simulink model "RM3_cHydraulic_PTO_WithSimscapeJustPiston"  (R2020b)
settings: Solver=ode4  StartTime=0  StopTime=400  FixedStep=0.001  MaxStep=0.001  RelTol=1e-3
values from neighbouring files (symbols this model uses):
  Apiston = 0.0378    [ptoSimInputFile.m]
  Vo_cylinder = 15*Apiston    (= 0.567)    [ptoSimInputFile.m]
undefined symbols (not defined in the file or in its folder): RM3_CHydraulic_resultsOriginal
libraries: fl_lib x13, nesl_utility x8, PTOSim_Lib x2, sh_lib x1
settings Model: Creator=jleonqu  LastModifiedBy=jleonqu
settings SolverCC: ZeroCrossControl=DisableAll  AutoInsertRateTranBlk=on
settings DataIOCC: ReturnWorkspaceOutputs=off
settings OptimizationCC: SimCompilerOptimization=on

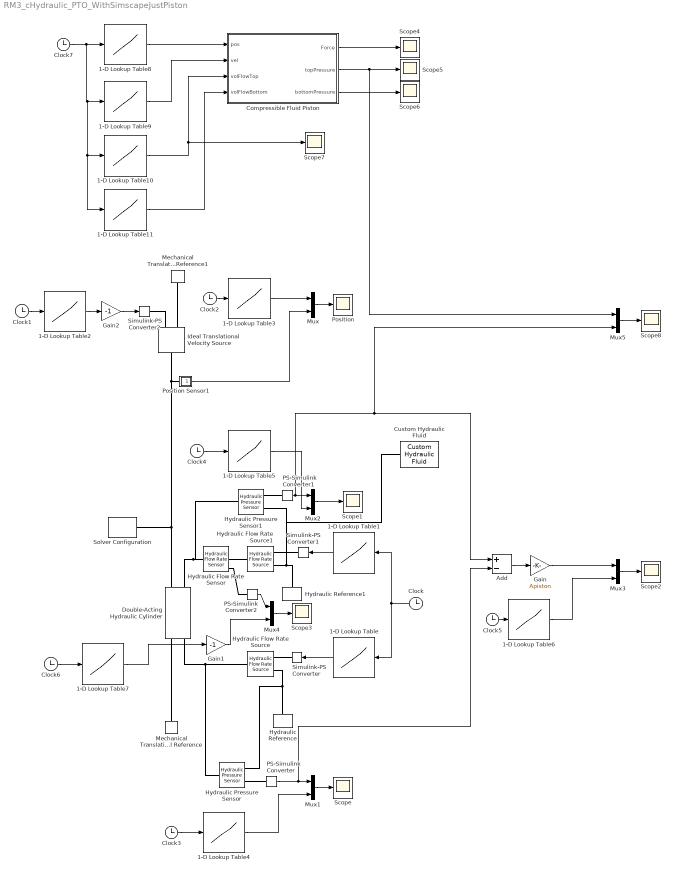
== system RM3_cHydraulic_PTO_WithSimscapeJustPiston ==
  1-D Lookup Table : Lookup_n-D  NumberOfTableDimensions=1  BreakpointsForDimension1=RM3_CHydraulic_resultsOriginal(:,1)  Table=RM3_CHydraulic_resultsOriginal(:,5)  InternalRulePriority=Speed  RndMeth=Simplest  InputSameDT=on
  1-D Lookup Table1 : Lookup_n-D  NumberOfTableDimensions=1  BreakpointsForDimension1=RM3_CHydraulic_resultsOriginal(:,1)  Table=RM3_CHydraulic_resultsOriginal(:,4)  InternalRulePriority=Speed  RndMeth=Simplest  InputSameDT=on
  1-D Lookup Table10 : Lookup_n-D  NumberOfTableDimensions=1  BreakpointsForDimension1=RM3_CHydraulic_resultsOriginal(:,1)  Table=RM3_CHydraulic_resultsOriginal(:,4)  InternalRulePriority=Speed  RndMeth=Simplest  InputSameDT=on
  1-D Lookup Table11 : Lookup_n-D  NumberOfTableDimensions=1  BreakpointsForDimension1=RM3_CHydraulic_resultsOriginal(:,1)  Table=RM3_CHydraulic_resultsOriginal(:,5)  InternalRulePriority=Speed  RndMeth=Simplest  InputSameDT=on
  1-D Lookup Table2 : Lookup_n-D  NumberOfTableDimensions=1  BreakpointsForDimension1=RM3_CHydraulic_resultsOriginal(:,1)  Table=RM3_CHydraulic_resultsOriginal(:,3)  InternalRulePriority=Speed  RndMeth=Simplest  InputSameDT=on
  1-D Lookup Table3 : Lookup_n-D  NumberOfTableDimensions=1  BreakpointsForDimension1=RM3_CHydraulic_resultsOriginal(:,1)  Table=RM3_CHydraulic_resultsOriginal(:,2)  InternalRulePriority=Speed  RndMeth=Simplest  InputSameDT=on
  1-D Lookup Table4 : Lookup_n-D  NumberOfTableDimensions=1  BreakpointsForDimension1=RM3_CHydraulic_resultsOriginal(:,1)  Table=RM3_CHydraulic_resultsOriginal(:,8)  InternalRulePriority=Speed  RndMeth=Simplest  InputSameDT=on
  1-D Lookup Table5 : Lookup_n-D  NumberOfTableDimensions=1  BreakpointsForDimension1=RM3_CHydraulic_resultsOriginal(:,1)  Table=RM3_CHydraulic_resultsOriginal(:,7)  InternalRulePriority=Speed  RndMeth=Simplest  InputSameDT=on
  1-D Lookup Table6 : Lookup_n-D  NumberOfTableDimensions=1  BreakpointsForDimension1=RM3_CHydraulic_resultsOriginal(:,1)  Table=RM3_CHydraulic_resultsOriginal(:,6)  InternalRulePriority=Speed  RndMeth=Simplest  InputSameDT=on
  1-D Lookup Table7 : Lookup_n-D  NumberOfTableDimensions=1  BreakpointsForDimension1=RM3_CHydraulic_resultsOriginal(:,1)  Table=RM3_CHydraulic_resultsOriginal(:,4)  InternalRulePriority=Speed  RndMeth=Simplest  InputSameDT=on
  1-D Lookup Table8 : Lookup_n-D  NumberOfTableDimensions=1  BreakpointsForDimension1=RM3_CHydraulic_resultsOriginal(:,1)  Table=RM3_CHydraulic_resultsOriginal(:,2)  InternalRulePriority=Speed  RndMeth=Simplest  InputSameDT=on
  1-D Lookup Table9 : Lookup_n-D  NumberOfTableDimensions=1  BreakpointsForDimension1=RM3_CHydraulic_resultsOriginal(:,1)  Table=RM3_CHydraulic_resultsOriginal(:,3)  InternalRulePriority=Speed  RndMeth=Simplest  InputSameDT=on
  Add : Sum  Inputs=+-
  Clock{,1..7} (8 alike) : Clock
  Compressible Fluid Piston : Subsystem
  Custom Hydraulic Fluid : fl_lib/Hydraulic/Hydraulic Utilities/Custom Hydraulic Fluid  density=850 kg/m^3  viscosity_kin=18e-6 m^2/s  bulk=1.86e9 Pa  alpha=0.005  range_error=2
      settings: SourceProductBaseCode=SS  InternalSimscapePortConfiguration="{\"Bottom\":[],\"Left\":[],\"Right\":[{\"id\":\"G\",\"label\":\"\",\"type\":\"foundation.hydraulic.hydraulic\"}],\"Top\":[]}"
  Double-Acting Hydraulic Cylinder : sh_lib/Hydraulic Cylinders/Double-Acting Hydraulic Cylinder  area_A=Apiston m^2  area_B=Apiston m^2  stroke=2*Vo_cylinder/Apiston m  init_pos=0.3*2*Vo_cylinder/Apiston m  dead_vol_A=1e-4 m^3  dead_vol_B=1e-4 m^3  init_pressure_A=2.1333e7 Pa  init_pressure_B=2.1333e7 Pa  k_sh=1.4  stiff=1e6 N/m  D=150 N/(m/s)  hardstop_model=1  transition=0.1 mm  or=1
      settings: SourceProductBaseCode=SH  InternalSimscapePortConfiguration="{\"Bottom\":[],\"Left\":[{\"id\":\"C\",\"label\":\"C\",\"type\":\"foundation.mechanical.translational.translational\"},{\"id\":\"A\",\"label\":\"A\",\"type\":\"foundation.hydraulic.hydraulic\"}],\"Right\":[{\"id\":\"R\",\"label\":\"R\",\"type\":\"foundation.mechanical.translational.translational\"},{\"id\":\"B\",\"label\":\"B\",\"type\":\"foundation.hydraulic.hydraulic\"}],\"Top\":[]}"
  Gain : Gain  Gain=Apiston
  Gain1 : Gain  Gain=-1
  Gain2 : Gain  Gain=-1
  Hydraulic Flow Rate Sensor : fl_lib/Hydraulic/Hydraulic Sensors/Hydraulic Flow Rate Sensor
  Hydraulic Flow Rate Source : fl_lib/Hydraulic/Hydraulic Sources/Hydraulic Flow Rate Source
      settings: SourceProductBaseCode=SS  InternalSimscapePortConfiguration="{\"Bottom\":[],\"Left\":[{\"id\":\"P\",\"label\":\"P\",\"type\":\"foundation.hydraulic.hydraulic\"}],\"Right\":[{\"id\":\"S\",\"label\":\"S\",\"type\":\"input\"},{\"id\":\"T\",\"label\":\"T\",\"type\":\"foundation.hydraulic.hydraulic\"}],\"Top\":[]}"
  Hydraulic Flow Rate Source1 : fl_lib/Hydraulic/Hydraulic Sources/Hydraulic Flow Rate Source
      settings: SourceProductBaseCode=SS  InternalSimscapePortConfiguration="{\"Bottom\":[],\"Left\":[{\"id\":\"P\",\"label\":\"P\",\"type\":\"foundation.hydraulic.hydraulic\"}],\"Right\":[{\"id\":\"S\",\"label\":\"S\",\"type\":\"input\"},{\"id\":\"T\",\"label\":\"T\",\"type\":\"foundation.hydraulic.hydraulic\"}],\"Top\":[]}"
  Hydraulic Pressure Sensor : fl_lib/Hydraulic/Hydraulic Sensors/Hydraulic Pressure Sensor
  Hydraulic Pressure Sensor1 : fl_lib/Hydraulic/Hydraulic Sensors/Hydraulic Pressure Sensor
  Hydraulic Reference : fl_lib/Hydraulic/Hydraulic Elements/Hydraulic Reference
  Hydraulic Reference1 : fl_lib/Hydraulic/Hydraulic Elements/Hydraulic Reference
  Ideal Translational Velocity Source : fl_lib/Mechanical/Mechanical Sources/Ideal Translational Velocity Source
  Mechanical Translational Reference : fl_lib/Mechanical/Translational Elements/Mechanical Translational Reference
  Mechanical Translational Reference1 : fl_lib/Mechanical/Translational Elements/Mechanical Translational Reference
  Mux{,1..5} (6 alike) : Mux  Inputs=2
  PS-Simulink Converter : nesl_utility/PS-Simulink Converter  PhysicalDomain=network_engine_domain  SubClassName=ps_output  LeftPortType=input  RightPortType=output  PseudoPeriodic=off  Frequencies=[]  Unit=inherit  AffineConversion=off
  PS-Simulink Converter1 : nesl_utility/PS-Simulink Converter  PhysicalDomain=network_engine_domain  SubClassName=ps_output  LeftPortType=input  RightPortType=output  PseudoPeriodic=off  Frequencies=[]  Unit=inherit  AffineConversion=off
  PS-Simulink Converter2 : nesl_utility/PS-Simulink Converter  PhysicalDomain=network_engine_domain  SubClassName=ps_output  LeftPortType=input  RightPortType=output  PseudoPeriodic=off  Frequencies=[]  Unit=inherit  AffineConversion=off
  Position : Scope
  Position Sensor1 : Subsystem
      mask Display: disp('P');
  Scope{,1..8} (9 alike) : Scope
  Simulink-PS Converter : nesl_utility/Simulink-PS Converter  PhysicalDomain=network_engine_domain  SubClassName=ps_input  LeftPortType=input  RightPortType=output  PseudoPeriodic=off  Frequencies=[]  NoiseDistribution=none  NoiseParameters=[]  Unit=1  AffineConversion=off  FilteringAndDerivatives=provide  SimscapeFilterOrder=1  InputFilterTimeConstant=0.001  UdotUserProvided=0
  Simulink-PS Converter1 : nesl_utility/Simulink-PS Converter  PhysicalDomain=network_engine_domain  SubClassName=ps_input  LeftPortType=input  RightPortType=output  PseudoPeriodic=off  Frequencies=[]  NoiseDistribution=none  NoiseParameters=[]  Unit=1  AffineConversion=off  FilteringAndDerivatives=provide  SimscapeFilterOrder=1  InputFilterTimeConstant=0.001  UdotUserProvided=0
  Simulink-PS Converter2 : nesl_utility/Simulink-PS Converter  PhysicalDomain=network_engine_domain  SubClassName=ps_input  LeftPortType=input  RightPortType=output  PseudoPeriodic=off  Frequencies=[]  NoiseDistribution=none  NoiseParameters=[]  Unit=1  AffineConversion=off  FilteringAndDerivatives=provide  SimscapeFilterOrder=1  InputFilterTimeConstant=0.001  UdotUserProvided=0
  Solver Configuration : nesl_utility/Solver Configuration  PhysicalDomain=network_engine_domain  SubClassName=solver  LeftPortType=input  RightPortType=generic  Tones=[]  Harmonics=[]  SimulateNoise=off  Profile=off  UseLocalSampling=off  EnableSwitchedLinearOptims=on  FrequencyDomain=off  UseCCode=off  RelTol=0.001  AbsTol=1e-06  MinStep=1e-09  ToWorkspace=off  RevertToSquareIcSolve=off  NumHomotopyIterations=100  PhasorMode=off  PhasorModeNumHarmonics=1  DoDC=off  ResidualTolerance=1e-09  UseLocalSolver=on  LocalSolverChoice=NE_BACKWARD_EULER_ADVANCER  LocalSolverSampleTime=0.001  DoFixedCost=on  MaxNonlinIter=3  MaxModeIter=2  ComputeImpulses=off  ImpulseIterations=2  LinearAlgebra=auto  EquationFormulation=NE_TIME_EF  DelaysMemoryBudget=1024  AutomaticFiltering=on  FilteringTimeConstant=0.001  PartitionStorageMethod=AS_NEEDED  PartitionMemoryBudget=1024  PartitionMethod=ROBUST
  wires:
  1-D Lookup Table/1 -> Simulink-PS Converter/1
  1-D Lookup Table1/1 -> Simulink-PS Converter1/1
  Clock/1 -> 1-D Lookup Table1/1, 1-D Lookup Table/1
  Clock1/1 -> 1-D Lookup Table2/1
  Clock2/1 -> 1-D Lookup Table3/1
  Mux/1 -> Position/1
  Position Sensor1/1(P) -> Mux/2
  1-D Lookup Table3/1 -> Mux/1
  PS-Simulink Converter/1 -> Add/2, Mux1/1
  1-D Lookup Table4/1 -> Mux1/2
  Mux1/1 -> Scope/1
  Clock3/1 -> 1-D Lookup Table4/1
  PS-Simulink Converter1/1 -> Mux5/2, Add/1, Mux2/1
  Clock4/1 -> 1-D Lookup Table5/1
  1-D Lookup Table5/1 -> Mux2/2
  Mux2/1 -> Scope1/1
  Add/1 -> Gain/1
  Clock5/1 -> 1-D Lookup Table6/1
  1-D Lookup Table6/1 -> Mux3/2
  Gain/1 -> Mux3/1
  Mux3/1 -> Scope2/1
  PS-Simulink Converter2/1 -> Mux4/1
  Mux4/1 -> Scope3/1
  Clock6/1 -> 1-D Lookup Table7/1
  1-D Lookup Table7/1 -> Gain1/1
  Gain1/1 -> Mux4/2
  1-D Lookup Table8/1 -> Compressible Fluid Piston/1(pos)
  1-D Lookup Table9/1 -> Compressible Fluid Piston/2(vel)
  Clock7/1 -> 1-D Lookup Table11/1, 1-D Lookup Table10/1, 1-D Lookup Table9/1, 1-D Lookup Table8/1
  1-D Lookup Table10/1 -> Scope7/1, Compressible Fluid Piston/3(volFlowTop)
  1-D Lookup Table11/1 -> Compressible Fluid Piston/4(volFlowBottom)
  Compressible Fluid Piston/1(Force) -> Scope4/1
  Compressible Fluid Piston/2(topPressure) -> Mux5/1, Scope5/1
  Compressible Fluid Piston/3(bottomPressure) -> Scope6/1
  Mux5/1 -> Scope8/1
  1-D Lookup Table2/1 -> Gain2/1
  Gain2/1 -> Simulink-PS Converter2/1
  connections:
  Hydraulic Flow Rate Source/LConn1 -- Hydraulic Pressure Sensor/LConn1 -- Double-Acting Hydraulic Cylinder/LConn2
  Hydraulic Pressure Sensor1/LConn1 -- Hydraulic Flow Rate Sensor/LConn1 -- Double-Acting Hydraulic Cylinder/RConn2
  Hydraulic Reference/LConn1 -- Hydraulic Flow Rate Source/RConn2 -- Hydraulic Pressure Sensor/RConn1
  Hydraulic Reference1/LConn1 -- Custom Hydraulic Fluid/RConn1 -- Hydraulic Pressure Sensor1/RConn1 -- Hydraulic Flow Rate Source1/RConn2
  Simulink-PS Converter/RConn1 -- Hydraulic Flow Rate Source/RConn1
  Simulink-PS Converter1/RConn1 -- Hydraulic Flow Rate Source1/RConn1
  Mechanical Translational Reference/LConn1 -- Double-Acting Hydraulic Cylinder/LConn1
  Ideal Translational Velocity Source/LConn1 -- Solver Configuration/RConn1 -- Double-Acting Hydraulic Cylinder/RConn1 -- Position Sensor1/LConn1
  Mechanical Translational Reference1/LConn1 -- Ideal Translational Velocity Source/RConn2
  Simulink-PS Converter2/RConn1 -- Ideal Translational Velocity Source/RConn1
  PS-Simulink Converter/LConn1 -- Hydraulic Pressure Sensor/RConn2
  PS-Simulink Converter1/LConn1 -- Hydraulic Pressure Sensor1/RConn2
  Hydraulic Flow Rate Sensor/RConn2 -- Hydraulic Flow Rate Source1/LConn1
  PS-Simulink Converter2/LConn1 -- Hydraulic Flow Rate Sensor/RConn1

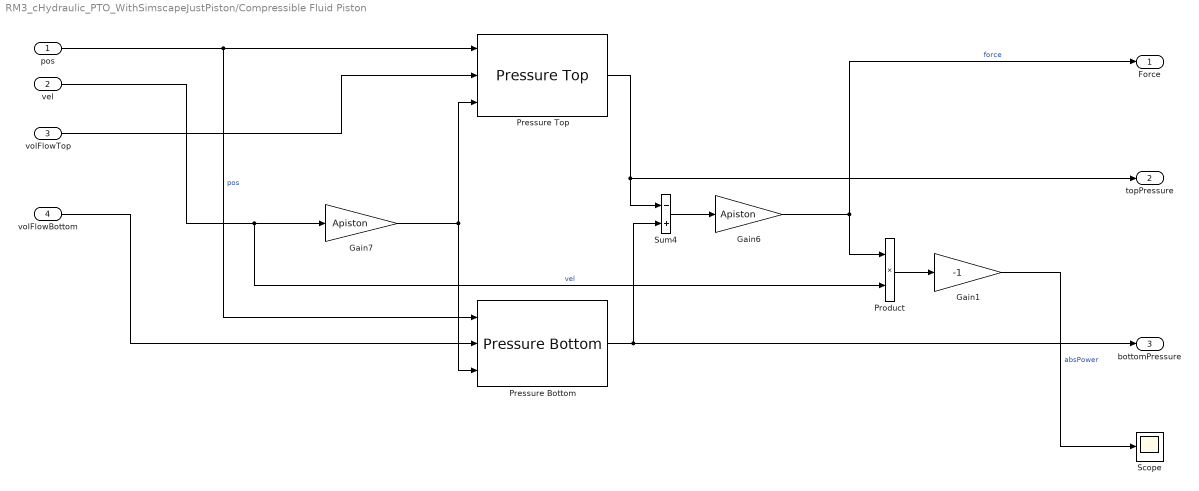
== system RM3_cHydraulic_PTO_WithSimscapeJustPiston/Compressible Fluid Piston ==
  pos : Inport
  vel : Inport  Port=2
  volFlowTop : Inport  Port=3
  volFlowBottom : Inport  Port=4
  Gain1 : Gain  Gain=-1
  Gain6 : Gain  Gain=Apiston
  Gain7 : Gain  Gain=Apiston
  Pressure Bottom : PTOSim_Lib/Hydraulic/Compressible Fluid Piston/Pressure Bottom  SystemSampleTime=-1  VariantActivationTime=update diagram  Latency=0  AutoFrameSizeCalculation=off
      link override Constant1: Value=Vo_cylinder
      link override Gain4: Gain=Beta_e
      link override Gain5: Gain=Apiston
      link override Integrator3: InitialCondition=2.1333e7
      settings: SourceProductName=PTO-Sim
  Pressure Top : PTOSim_Lib/Hydraulic/Compressible Fluid Piston/Pressure Top  SystemSampleTime=-1  VariantActivationTime=update diagram  Latency=0  AutoFrameSizeCalculation=off
      link override Constant: Value=Vo_cylinder
      link override Gain1: Gain=Beta_e
      link override Gain2: Gain=Apiston
      link override Integrator2: InitialCondition=2.1333e7
      settings: SourceProductName=PTO-Sim
  Product : Product
  Scope : Scope
  Sum4 : Sum  Inputs=-+
  Force : Outport
  topPressure : Outport  Port=2
  bottomPressure : Outport  Port=3
  wires:
  Product/1 -> Gain1/1
  Pressure Bottom/1 -> bottomPressure/1, Sum4/2
  vel/1 -> Gain7/1, Product/2  "vel"
  Gain7/1 -> Pressure Top/3, Pressure Bottom/3
  Gain1/1 -> Scope/1  "absPower"
  Gain6/1 -> Force/1, Product/1  "force"
  volFlowBottom/1 -> Pressure Bottom/2
  volFlowTop/1 -> Pressure Top/2
  pos/1 -> Pressure Top/1, Pressure Bottom/1  "pos"
  Pressure Top/1 -> topPressure/1, Sum4/1
  Sum4/1 -> Gain6/1

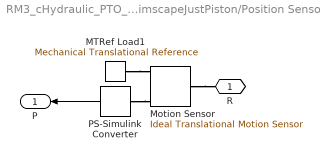
== system RM3_cHydraulic_PTO_WithSimscapeJustPiston/Position Sensor1 ==
  MTRef Load1 : fl_lib/Mechanical/Translational Elements/Mechanical Translational Reference  Tag=Factory Generic
  Motion Sensor : fl_lib/Mechanical/Mechanical Sensors/Ideal Translational Motion Sensor  offset=0 m
  PS-Simulink Converter : nesl_utility/PS-Simulink Converter  PhysicalDomain=network_engine_domain  SubClassName=ps_output  LeftPortType=input  RightPortType=output  PseudoPeriodic=off  Frequencies=[]  Unit=1  AffineConversion=off
  R : PMIOPort  Side=Left
  P : Outport  VectorParamsAs1DForOutWhenUnconnected=off
  wires:
  PS-Simulink Converter/1 -> P/1
  connections:
  PS-Simulink Converter/LConn1 -- Motion Sensor/RConn3
  Motion Sensor/LConn1 -- R/RConn1
  MTRef Load1/LConn1 -- Motion Sensor/RConn1
